simulink model "assignment_1"  (R2020b)
settings: Solver=VariableStepAuto  StartTime=0.0  StopTime=200  RelTol=1e-3
settings Model: Creator=Sudhanshu  LastModifiedBy=Sudhanshu

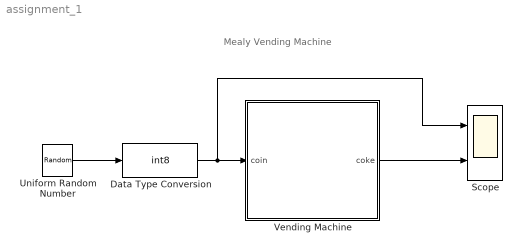
== system assignment_1 ==
  note: Mealy Vending Machine
  Data Type Conversion : DataTypeConversion  OutDataTypeStr=int8  RndMeth=Nearest  SaturateOnIntegerOverflow=on
  Scope : Scope  NumInputPorts=2
  Uniform Random Number : UniformRandomNumber  Minimum=0  Maximum=2  Seed=300  SampleTime=10
  Vending Machine : Stateflow chart  TreatAsAtomicUnit=on
  wires:
  Uniform Random Number/1 -> Data Type Conversion/1
  Data Type Conversion/1 -> Scope/1, Vending Machine/1(coin)
  Vending Machine/1(coke) -> Scope/2

== stateflow chart assignment_1/Vending Machine ==
  settings: stateMachineType=MEALY_MACHINE  initializeOutput=1
  state money_0
  state nickel_recieved
  state dime_recieved
  money_0 -> nickel_recieved [order 1] : [coin==1]{coke=0}
  nickel_recieved -> money_0 [order 2] : [coin==2]{coke=1}
  (default) -> money_0
  dime_recieved -> money_0 [order 1] : [coin==1]{coke=1}
  money_0 -> dime_recieved [order 2] : [coin==2]{coke=0}
  nickel_recieved -> dime_recieved [order 1] : [coin==1]{coke=0}
  dime_recieved -> nickel_recieved [order 2] : [coin==2]{coke=1}
  data: coin input; coke output double
